simulink model "BasicWithOFDM"  (R2014b)
settings: Solver=VariableStepDiscrete  StartTime=0.0  StopTime=20.0  RelTol=1e-3
PreLoadFcn:
  | loadvar
libraries: commcnvcod2 x4, dspsigops x4, commdigbbndam3 x4, commofdm x2, commchan3 x1, commrandsrc2 x1, commsink2 x1
settings Model: Creator=yz10g11  LastModifiedBy=Yuan
settings DataIOCC: ExternalInput=[0 0 0 1 0]'
settings DebuggingCC: UnderspecifiedInitializationDetection=Classic  MergeDetectMultiDrivingBlocksExec=none

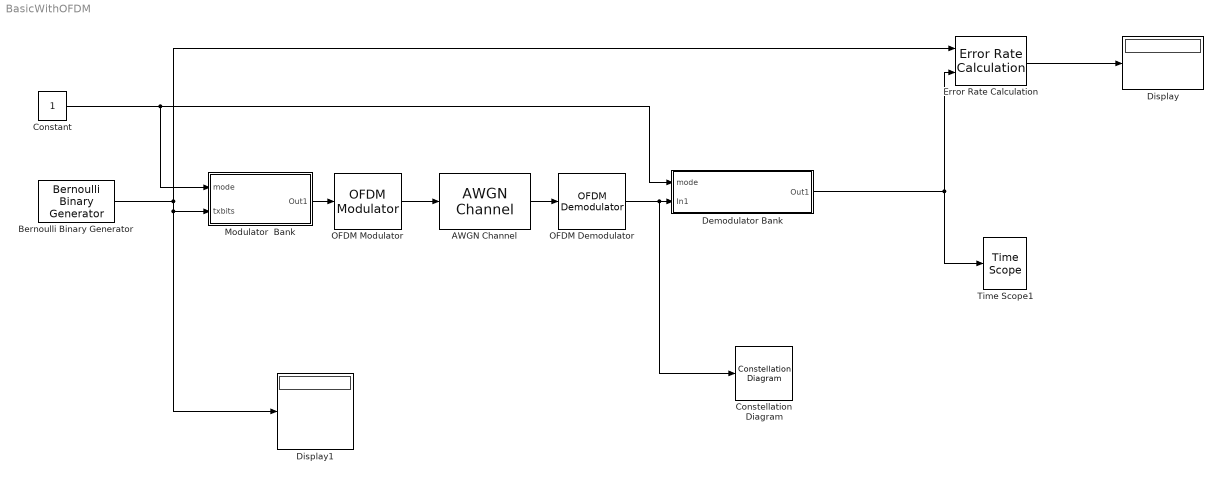
== system BasicWithOFDM ==
  AWGN Channel : commchan3/AWGN Channel  InputProcessing=Columns as channels (frame based)  seed=67  noiseMode="Signal to noise ratio  (Eb/No)"  EbNodB=30  EsNodB=10  SNRdB=10  bitsPerSym=1  Ps=1  Tsym=2  variance=1
  Bernoulli Binary Generator : commrandsrc2/Bernoulli Binary Generator  P=0.5  seed=911  Ts=1  frameBased=on  sampPerFrame=4  orient=off  outDataType=boolean
  Constant : Constant
  Constellation Diagram : ConstellationDiagram
  "Demodulator Bank " : Subsystem
  Display : Display
  Display1 : Display
  Error Rate Calculation : commsink2/Error Rate Calculation  N=10  st_delay=0  cp_mode=Entire frame  subframe=[]  PMode=Port  WsName=ErrorVec  RsMode2=off  stop=off  numErr=100  maxBits=1e6
  "Modulator  Bank " : Subsystem
  OFDM Demodulator : commofdm/OFDM Demodulator  SimulateUsing=Interpreted execution  FFTLength=8  NumGuardBandCarriers=[3; 3]  RemoveDCCarrier=off  PilotOutputPort=off  PilotCarrierIndices=[12; 26; 40; 54]  CyclicPrefixLength=2  NumSymbols=1  NumReceiveAntennas=1
  OFDM Modulator : commofdm/OFDM Modulator  SimulateUsing=Interpreted execution  FFTLength=8  NumGuardBandCarriers=[3; 3]  InsertDCNull=off  PilotInputPort=off  PilotCarrierIndices=[12; 26; 40; 54]  CyclicPrefixLength=2  Windowing=off  WindowLength=1  NumSymbols=1  NumTransmitAntennas=1
  Time Scope1 : TimeScope  DefaultConfigurationName=spbscopes.TimeScopeBlockCfg
  wires:
  Error Rate Calculation/1 -> Display/1
  "Demodulator Bank "/1(Out1) -> Time Scope1/1, Error Rate Calculation/2
  Bernoulli Binary Generator/1 -> Display1/1, "Modulator  Bank "/2("txbits "), Error Rate Calculation/1
  Constant/1 -> "Demodulator Bank "/1("mode "), "Modulator  Bank "/1("mode ")
  "Modulator  Bank "/1(Out1) -> OFDM Modulator/1
  OFDM Modulator/1 -> AWGN Channel/1
  AWGN Channel/1 -> OFDM Demodulator/1
  OFDM Demodulator/1 -> Constellation Diagram/1, "Demodulator Bank "/2(In1)

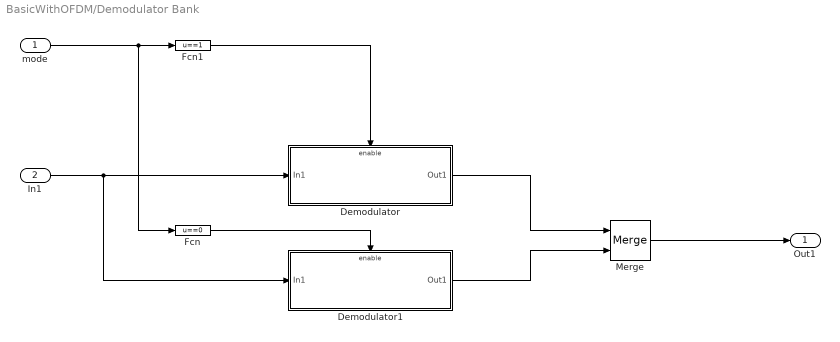
== system BasicWithOFDM/Demodulator Bank  ==
  "mode " : Inport
  In1 : Inport  Port=2
  Demodulator : Subsystem
  Demodulator1 : Subsystem
  Fcn : Fcn  Expr=u==0
  Fcn1 : Fcn  Expr=u==1
  Merge : Merge
  Out1 : Outport
  wires:
  In1/1 -> Demodulator1/1(In1), Demodulator/1(In1)
  "mode "/1 -> Fcn/1, Fcn1/1
  Fcn1/1 -> Demodulator/Enable
  Fcn/1 -> Demodulator1/Enable
  Demodulator/1(Out1) -> Merge/1
  Demodulator1/1(Out1) -> Merge/2
  Merge/1 -> Out1/1

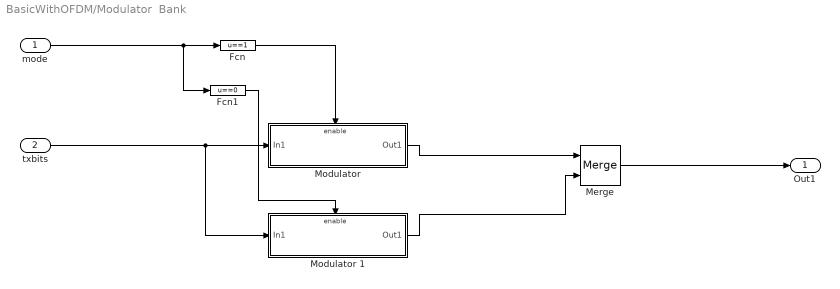
== system BasicWithOFDM/Modulator  Bank  ==
  "mode " : Inport
  "txbits " : Inport  Port=2
  Fcn : Fcn  Expr=u==1
  Fcn1 : Fcn  Expr=u==0
  Merge : Merge
  "Modulator " : Subsystem
  Modulator 1 : Subsystem
  Out1 : Outport
  wires:
  "mode "/1 -> Fcn1/1, Fcn/1
  Fcn/1 -> "Modulator "/Enable
  Fcn1/1 -> Modulator 1/Enable
  "Modulator "/1(Out1) -> Merge/1
  Modulator 1/1(Out1) -> Merge/2
  Merge/1 -> Out1/1
  "txbits "/1 -> Modulator 1/1(In1), "Modulator "/1(In1)

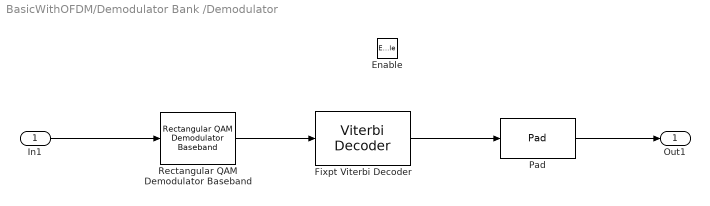
== system BasicWithOFDM/Demodulator Bank /Demodulator ==
  In1 : Inport
  Enable : EnablePort
  Fixpt Viterbi Decoder : commcnvcod2/Viterbi Decoder  trellis=poly2trellis(9, [561 753])  isPunctured=off  punctureVector=[1 1 0 1 1 0].'  erasures=off  dectype=Hard decision  runSigValErrCheck=off  nsdecb=3  smWordLength=16  tbdepth=Traceback_depth  opmode=Continuous  reset=off  outDataType=boolean  delayedResetAction=off
  Pad : dspsigops/Pad  padAlong=Columns  dimsToPad=1  valSrc=Specify via dialog  padVal=0  spec=Output size  padNumOutRowsSpecMethod=User-specified  numOutRows=4  padNumOutColsSpecMethod=User-specified  numOutCols=1  isVarDimsMode=off  padBeginning=0  padEnd=0  outSizeMode=User-specified  outSize=1  padSigAt=End  trunc_flag=None  roundingMode=Floor  overflowMode=off  truncOrWrapMode=Truncate  wrap_flag=None
  Rectangular QAM Demodulator Baseband : commdigbbndam3/Rectangular QAM Demodulator Baseband  M=16  PowType=Min. distance between symbols  MinDist=2  AvgPow=1  PeakPow=1  Ph=0  Dec=Gray  Mapping=[0:15]  OutType=Bit  DecType=Hard decision  VarSource=Dialog  Variance=1  outDtype1=uint8  outDtype2=Inherit via internal rule  derotateFactorWordLen=16  denormFactorWordLen=16  prodOutWordLen=32  prodOutRoundingMode=Floor  prodOutOverflowMode=Wrap  sumWordLen=32
  Out1 : Outport
  wires:
  In1/1 -> Rectangular QAM Demodulator Baseband/1
  Rectangular QAM Demodulator Baseband/1 -> Fixpt Viterbi Decoder/1
  Fixpt Viterbi Decoder/1 -> Pad/1
  Pad/1 -> Out1/1

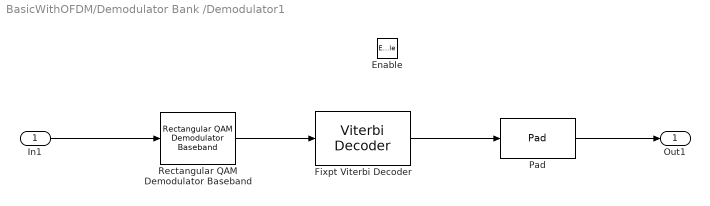
== system BasicWithOFDM/Demodulator Bank /Demodulator1 ==
  In1 : Inport
  Enable : EnablePort
  Fixpt Viterbi Decoder : commcnvcod2/Viterbi Decoder  trellis=poly2trellis(9, [561 753])  isPunctured=off  punctureVector=[1 1 0 1 1 0].'  erasures=off  dectype=Hard decision  runSigValErrCheck=off  nsdecb=3  smWordLength=16  tbdepth=Traceback_depth  opmode=Continuous  reset=off  outDataType=boolean  delayedResetAction=off
  Pad : dspsigops/Pad  padAlong=Columns  dimsToPad=1  valSrc=Specify via dialog  padVal=0  spec=Output size  padNumOutRowsSpecMethod=User-specified  numOutRows=4  padNumOutColsSpecMethod=User-specified  numOutCols=1  isVarDimsMode=off  padBeginning=0  padEnd=0  outSizeMode=User-specified  outSize=1  padSigAt=End  trunc_flag=None  roundingMode=Floor  overflowMode=off  truncOrWrapMode=Truncate  wrap_flag=None
  Rectangular QAM Demodulator Baseband : commdigbbndam3/Rectangular QAM Demodulator Baseband  M=4  PowType=Min. distance between symbols  MinDist=2  AvgPow=1  PeakPow=1  Ph=0  Dec=Gray  Mapping=[0:15]  OutType=Bit  DecType=Hard decision  VarSource=Dialog  Variance=1  outDtype1=uint8  outDtype2=Inherit via internal rule  derotateFactorWordLen=16  denormFactorWordLen=16  prodOutWordLen=32  prodOutRoundingMode=Floor  prodOutOverflowMode=Wrap  sumWordLen=32
  Out1 : Outport
  wires:
  Pad/1 -> Out1/1
  Fixpt Viterbi Decoder/1 -> Pad/1
  Rectangular QAM Demodulator Baseband/1 -> Fixpt Viterbi Decoder/1
  In1/1 -> Rectangular QAM Demodulator Baseband/1

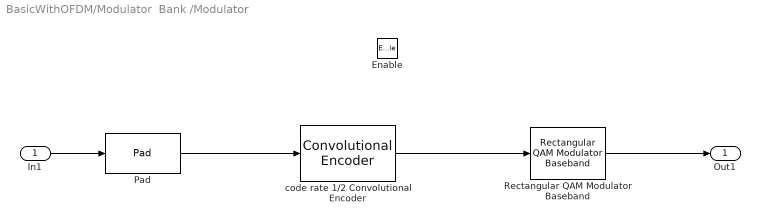
== system BasicWithOFDM/Modulator  Bank /Modulator  ==
  In1 : Inport
  Enable : EnablePort
  Pad : dspsigops/Pad  padAlong=Columns  dimsToPad=1  valSrc=Specify via dialog  padVal=0  spec=Output size  padNumOutRowsSpecMethod=User-specified  numOutRows=4  padNumOutColsSpecMethod=User-specified  numOutCols=1  isVarDimsMode=off  padBeginning=0  padEnd=0  outSizeMode=User-specified  outSize=1  padSigAt=End  trunc_flag=None  roundingMode=Floor  overflowMode=off  truncOrWrapMode=Truncate  wrap_flag=None
  Rectangular QAM Modulator Baseband : commdigbbndam3/Rectangular QAM Modulator Baseband  M=16  InType=Bit  Enc=Gray  Mapping=[0:15]  PowType=Min. distance between symbols  MinDist=2  AvgPow=1  PeakPow=1  Ph=0  outDtype=double  outWordLen=16  outUDDataType=sfix(16)  outFracLenMode=Best precision  outFracLen=15
  code rate 1/2 Convolutional Encoder : commcnvcod2/Convolutional Encoder  trellis=poly2trellis(9, [561 753])  opMode=Continuous  DelayedResetAction=off  hasIniStPort=off  hasFinStPort=off  usePuncVector=off  punctureVector=[1 1 0 1 1 0].'  reset=Unused parameter value
  Out1 : Outport
  wires:
  Rectangular QAM Modulator Baseband/1 -> Out1/1
  code rate 1/2 Convolutional Encoder/1 -> Rectangular QAM Modulator Baseband/1
  In1/1 -> Pad/1
  Pad/1 -> code rate 1/2 Convolutional Encoder/1

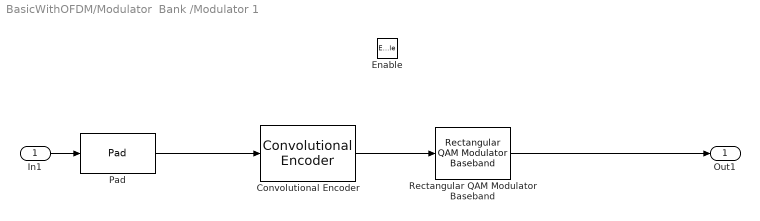
== system BasicWithOFDM/Modulator  Bank /Modulator 1 ==
  In1 : Inport
  Enable : EnablePort
  Convolutional Encoder : commcnvcod2/Convolutional Encoder  trellis=poly2trellis(9, [561 753])  opMode=Continuous  DelayedResetAction=off  hasIniStPort=off  hasFinStPort=off  usePuncVector=off  punctureVector=[1 1 0 1 1 0].'  reset=Unused parameter value
  Pad : dspsigops/Pad  padAlong=Columns  dimsToPad=1  valSrc=Specify via dialog  padVal=0  spec=Output size  padNumOutRowsSpecMethod=User-specified  numOutRows=2  padNumOutColsSpecMethod=User-specified  numOutCols=1  isVarDimsMode=off  padBeginning=0  padEnd=0  outSizeMode=User-specified  outSize=1  padSigAt=End  trunc_flag=None  roundingMode=Floor  overflowMode=off  truncOrWrapMode=Truncate  wrap_flag=None
  Rectangular QAM Modulator Baseband : commdigbbndam3/Rectangular QAM Modulator Baseband  M=4  InType=Bit  Enc=Gray  Mapping=[0:15]  PowType=Min. distance between symbols  MinDist=2  AvgPow=1  PeakPow=1  Ph=0  outDtype=double  outWordLen=16  outUDDataType=sfix(16)  outFracLenMode=Best precision  outFracLen=15
  Out1 : Outport
  wires:
  Convolutional Encoder/1 -> Rectangular QAM Modulator Baseband/1
  Rectangular QAM Modulator Baseband/1 -> Out1/1
  In1/1 -> Pad/1
  Pad/1 -> Convolutional Encoder/1
